simulink model "Wireless_Simulation_83kHz"  (R2013a)
settings: Solver=ode45  StartTime=0.0  StopTime=0.1  FixedStep=1e-6  RelTol=1e-3
libraries: powerlib x26
settings Model: Creator=pc  LastModifiedBy=pc

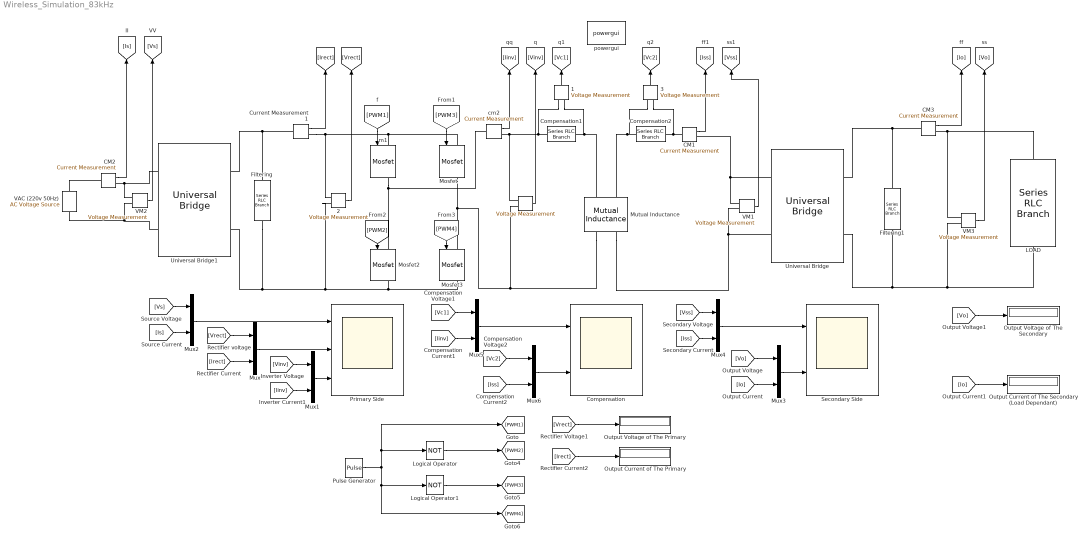
== system Wireless_Simulation_83kHz ==
   {,1..3} (4 alike) : powerlib/Measurements/Voltage Measurement  PhasorSimulation=off  OutputType=Complex  PSBequivalent=0
  CM1 : powerlib/Measurements/Current Measurement  PhasorSimulation=off  OutputType=Complex  PSBequivalent=0
  CM2 : powerlib/Measurements/Current Measurement  PhasorSimulation=off  OutputType=Complex  PSBequivalent=0
  CM3 : powerlib/Measurements/Current Measurement  PhasorSimulation=off  OutputType=Complex  PSBequivalent=0
  Compensation : Scope  NumInputPorts=2
      settings: ShowLegends=on  TimeRange=0.006000000000000005  YMin=-1000~-700  YMax=400~700  SaveName=ScopeData2
  Compensation1 : powerlib/Elements/Series RLC Branch  LConnTagsString=__new0  RConnTagsString=__new0  BranchType=C  Resistance=5  Inductance=268e-6  SetiL0=off  InitialCurrent=0  Capacitance=34.9e-9  Setx0=off  InitialVoltage=0  Measurements=None
  Compensation2 : powerlib/Elements/Series RLC Branch  LConnTagsString=__new0  RConnTagsString=__new0  BranchType=C  Resistance=0.1  Inductance=10e-3  SetiL0=off  InitialCurrent=0  Capacitance=34.6897e-9  Setx0=off  InitialVoltage=0  Measurements=None
  Current Measurement1 : powerlib/Measurements/Current Measurement  PhasorSimulation=off  OutputType=Complex  PSBequivalent=0
  Filtering : powerlib/Elements/Series RLC Branch  LConnTagsString=__new0  RConnTagsString=__new0  BranchType=C  Resistance=1e9  Inductance=1e-3  SetiL0=off  InitialCurrent=0  Capacitance=4400e-6  Setx0=off  InitialVoltage=0  Measurements=None
  Filtering1 : powerlib/Elements/Series RLC Branch  LConnTagsString=__new0  RConnTagsString=__new0  BranchType=C  Resistance=200  Inductance=1e-3  SetiL0=off  InitialCurrent=0  Capacitance=1600e-6  Setx0=off  InitialVoltage=0  Measurements=None
  LOAD : powerlib/Elements/Series RLC Branch  LConnTagsString=__new0  RConnTagsString=__new0  BranchType=R  Resistance=5.3  Inductance=10e-3  SetiL0=off  InitialCurrent=0  Capacitance=28e-9  Setx0=off  InitialVoltage=0  Measurements=None
  Logical Operator : Logic  Operator=NOT  AllPortsSameDT=off  OutDataTypeStr=boolean
  Logical Operator1 : Logic  Operator=NOT  AllPortsSameDT=off  OutDataTypeStr=boolean
  Mosfet : powerlib/Power Electronics/Mosfet  Ron=0.1  Lon=0  Rd=0.01  Vfd=0  IC=0  Rs=1e5  Cs=inf  Measurements=on
  Mosfet2 : powerlib/Power Electronics/Mosfet  Ron=0.1  Lon=0  Rd=0.01  Vfd=0  IC=0  Rs=1e5  Cs=inf  Measurements=on
  Mosfet3 : powerlib/Power Electronics/Mosfet  Ron=0.1  Lon=0  Rd=0.01  Vfd=0  IC=0  Rs=1e5  Cs=inf  Measurements=on
  Mutual Inductance : powerlib/Elements/Mutual Inductance  LConnTagsString=a|b  RConnTagsString=A|B  TypeOfMutual=Two or three windings with equal mutual terms  NumberOfWindings=2  SelfImpedance1=[0.12 100.452e-06]  SelfImpedance2=[ 0.12 101.065225e-06]  ThreeWindings=off  SelfImpedance3=[ 1.1 1.1e-03]  MutualImpedance=[0.1 13.315217e-6]  InductanceMatrix="[110.877 14 ;  14 110.877 ] * 1e-6"  ResistanceMatrix="[0.00697 0.1 ;  0.1 0.00697 ]"  Measurements=None
      settings: AttributesFormatString=\n
  Mux{,1..6} (7 alike) : Mux  Inputs=2
  Output Current of The Primary : Display
  Output Current of The Secondary (Load Dependant) : Display
  Output Voltage of The Primary : Display
  Output Voltage of The Secondary : Display
  Primary Side : Scope  NumInputPorts=3
      settings: ShowLegends=on  TimeRange=0.006000000000000005  YMin=-250~-25~-350  YMax=350~325~350
  Pulse Generator : DiscretePulseGenerator  PulseType=Time based  Period=1/85000  PulseWidth=10
  Secondary Side : Scope  NumInputPorts=2
      settings: ShowLegends=on  TimeRange=0.0006000000000000033  YMin=-2500~2.89611182090357  YMax=2500~13.8369786998723
  Universal Bridge : powerlib/Power Electronics/Universal Bridge  Arms=2  SnubberResistance=1e5  SnubberCapacitance=inf  Device=Diodes  Ron=1e-3  Lon=0  ForwardVoltages="[  0  0  ]"  ForwardVoltage=0  GTOparameters=[ 10e-6 , 20e-6 ]  IGBTparameters=[ 1e-6 , 2e-6 ]  Measurements=None  Measurements_2=None  converterType=Rectifier
  Universal Bridge1 : powerlib/Power Electronics/Universal Bridge  Arms=2  SnubberResistance=1e5  SnubberCapacitance=inf  Device=Diodes  Ron=1e-3  Lon=0  ForwardVoltages="[  0  0  ]"  ForwardVoltage=0  GTOparameters=[ 10e-6 , 20e-6 ]  IGBTparameters=[ 1e-6 , 2e-6 ]  Measurements=None  Measurements_2=None  converterType=Rectifier
  VAC (220v 50Hz) : powerlib/Electrical Sources/AC Voltage Source  Amplitude=311.175  Phase=0  Frequency=85000  SampleTime=0  Measurements=None
  VM1 : powerlib/Measurements/Voltage Measurement  PhasorSimulation=off  OutputType=Complex  PSBequivalent=0
  VM2 : powerlib/Measurements/Voltage Measurement  PhasorSimulation=off  OutputType=Complex  PSBequivalent=0
  VM3 : powerlib/Measurements/Voltage Measurement  PhasorSimulation=off  OutputType=Complex  PSBequivalent=0
  cm2 : powerlib/Measurements/Current Measurement  PhasorSimulation=off  OutputType=Complex  PSBequivalent=0
  m1 : powerlib/Power Electronics/Mosfet  Ron=0.1  Lon=0  Rd=0.01  Vfd=0  IC=0  Rs=1e5  Cs=inf  Measurements=on
  powergui : powerlib/powergui  Priority=1  SimulationMode=Continuous  SolverType=Tustin  SampleTime=1e-7  frequency=60  SPID=on  DisableSnubberDevices=on  DisableRonSwitches=off  DisableVfSwitches=off  SwTol=0  Interpol=off  DisplayEquations=off  frequencyindice=85000  Pbase=100e6  ErrMax=1e-4  Iterations=50  UnitsV=kV  UnitsW=MW  FunctionMessages=off  echomessages=off  HookPort=off  EnableUseOfTLC=off  x0status=blocks  RestoreLinks=warning  ResistiveCurrentMeasurement=off  Frange=[0:2:500]  Ylog=off  Xlog=on  ShowGrid=off  save=off  variable=ZData  ZoomFFT=off  StartTime=0.0  cycles=1  DisplayStyle=1  fundamental=60  FreqAxis=off  MaxFrequency=1000  frequencyindicesteady=1  RmsSteady=1  display=off  Ts=0  methode=off
  wires:
  [Vrect] -> Mux/1
  [Irect] -> Mux/2
  [Vinv] -> Mux1/1
  [Iinv] -> Mux1/2
  CM2/1 -> [Is]
  VM2/1 -> [Vs]
  [Vs] -> Mux2/1
  [Is] -> Mux2/2
  Mux2/1 -> Primary Side/1
  Mux/1 -> Primary Side/2
  Mux1/1 -> Primary Side/3
  [Vo] -> Mux3/1
  [Io] -> Mux3/2
  [Vss] -> Mux4/1
  [Iss] -> Mux4/2
  Mux4/1 -> Secondary Side/1
  Mux3/1 -> Secondary Side/2
  CM1/1 -> [Iss]
  [Vo] -> Output Voltage of The Secondary/1
  [Io] -> Output Current of The Secondary (Load Dependant)/1
  [PWM2] -> Mosfet2/1
  Logical Operator1/1 -> [PWM3]
  Logical Operator/1 -> [PWM2]
  [PWM4] -> Mosfet3/1
  [PWM3] -> Mosfet/1
  [PWM1] -> m1/1
  Pulse Generator/1 -> Logical Operator1/1, [PWM4], Logical Operator/1, [PWM1]
  Current Measurement1/1 -> [Irect]
  " 2"/1 -> [Vrect]
  VM1/1 -> [Vss]
  CM3/1 -> [Io]
  VM3/1 -> [Vo]
  cm2/1 -> [Iinv]
  " "/1 -> [Vinv]
  [Vrect] -> Output Voltage of The Primary/1
  [Irect] -> Output Current of The Primary/1
  " 1"/1 -> [Vc1]
  " 3"/1 -> [Vc2]
  [Vc1] -> Mux5/1
  [Iinv] -> Mux5/2
  [Vc2] -> Mux6/1
  [Iss] -> Mux6/2
  Mux5/1 -> Compensation/1
  Mux6/1 -> Compensation/2
  connections:
  Compensation2/LConn1 -- " 3"/LConn1 -- Mutual Inductance/LConn2
  CM2/RConn1 -- VM2/LConn1 -- Universal Bridge1/LConn1
  Mutual Inductance/RConn1 -- " "/LConn2 -- Mosfet/RConn1 -- Mosfet3/LConn1
  Universal Bridge/RConn1 -- CM3/LConn1 -- Filtering1/LConn1
  VM3/LConn2 -- Filtering1/RConn1 -- Universal Bridge/RConn2 -- LOAD/RConn1
  VM3/LConn1 -- LOAD/LConn1 -- CM3/RConn1
  Universal Bridge1/LConn2 -- VAC (220v 50Hz)/LConn1 -- VM2/LConn2
  Compensation2/RConn1 -- " 3"/LConn2 -- CM1/LConn1
  m1/RConn1 -- cm2/LConn1 -- Mosfet2/LConn1
  " "/LConn1 -- " 1"/LConn1 -- Compensation1/LConn1 -- cm2/RConn1
  Mutual Inductance/LConn1 -- " 1"/LConn2 -- Compensation1/RConn1
  VM1/LConn1 -- Universal Bridge/LConn1 -- CM1/RConn1
  Filtering/LConn1 -- Current Measurement1/LConn1 -- Universal Bridge1/RConn1
  Current Measurement1/RConn1 -- Mosfet/LConn1 -- m1/LConn1 -- " 2"/LConn1
  Mosfet3/RConn1 -- Filtering/RConn1 -- Universal Bridge1/RConn2 -- " 2"/LConn2 -- Mosfet2/RConn1
  Mutual Inductance/RConn2 -- VM1/LConn2 -- Universal Bridge/LConn2
  CM2/LConn1 -- VAC (220v 50Hz)/RConn1
